simulink model "Model_compare_SLX"  (R2019b)
settings: Solver=VariableStepAuto  StartTime=0.0  StopTime=100.0  RelTol=1e-3
undefined symbols (not defined in the file): Ts, x0_dyn, x0_kin
settings Model: Creator=djtn  LastModifiedBy=alber
settings SFSimCC: CustomCodeUndefinedFunction=UseInterfaceOnly
settings ConfigComp: DVModelCoverageObjectives=MCDC  DVTestSuiteOptimization=Auto  DVDetectOutOfBounds=on  DVRebuildModelRepresentation=Always

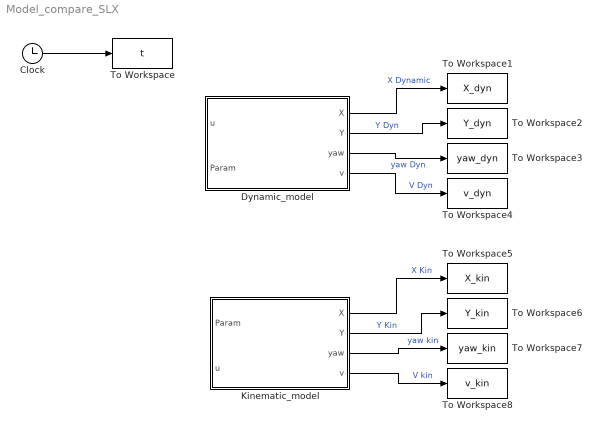
== system Model_compare_SLX ==
  Clock : Clock
  Dynamic_model : Subsystem
  Kinematic_model : Subsystem  TreatAsAtomicUnit=on
  To Workspace : ToWorkspace  VariableName=t  SampleTime=Ts
  To Workspace1 : ToWorkspace  VariableName=X_dyn  SampleTime=-1
  To Workspace2 : ToWorkspace  VariableName=Y_dyn  SampleTime=-1
  To Workspace3 : ToWorkspace  VariableName=yaw_dyn  SampleTime=-1
  To Workspace4 : ToWorkspace  VariableName=v_dyn  SampleTime=-1
  To Workspace5 : ToWorkspace  VariableName=X_kin  SampleTime=-1
  To Workspace6 : ToWorkspace  VariableName=Y_kin  SampleTime=-1
  To Workspace7 : ToWorkspace  VariableName=yaw_kin  SampleTime=-1
  To Workspace8 : ToWorkspace  VariableName=v_kin  SampleTime=-1
  wires:
  Clock/1 -> To Workspace/1
  Dynamic_model/1(X) -> To Workspace1/1  "X Dynamic"
  Dynamic_model/2(Y) -> To Workspace2/1  "Y Dyn"
  Dynamic_model/3(yaw) -> To Workspace3/1  "yaw Dyn"
  Dynamic_model/4(v) -> To Workspace4/1  "V Dyn"
  Kinematic_model/1(X) -> To Workspace5/1  "X Kin"
  Kinematic_model/2(Y) -> To Workspace6/1  "Y Kin"
  Kinematic_model/3(yaw) -> To Workspace7/1  "yaw kin"
  Kinematic_model/4(v) -> To Workspace8/1  "V kin"

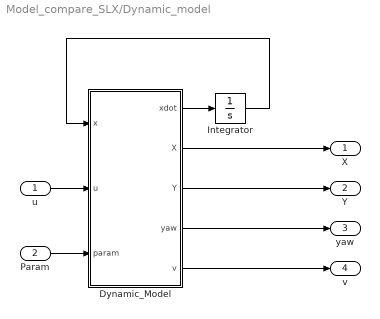
== system Model_compare_SLX/Dynamic_model ==
  u : Inport
  Param : Inport  Port=2
  Dynamic_Model : MATLAB Function  TreatAsAtomicUnit=on
  Integrator : Integrator  InitialCondition=x0_dyn
  X : Outport  PortDimensions=1  VectorParamsAs1DForOutWhenUnconnected=off
  Y : Outport  Port=2  PortDimensions=1  VectorParamsAs1DForOutWhenUnconnected=off
  yaw : Outport  Port=3  PortDimensions=1  VectorParamsAs1DForOutWhenUnconnected=off
  v : Outport  Port=4  PortDimensions=1  VectorParamsAs1DForOutWhenUnconnected=off
  wires:
  Integrator/1 -> Dynamic_Model/1(x)
  Dynamic_Model/1(xdot) -> Integrator/1
  u/1 -> Dynamic_Model/2(u)
  Dynamic_Model/2(X) -> X/1
  Dynamic_Model/3(Y) -> Y/1
  Dynamic_Model/4(yaw) -> yaw/1
  Dynamic_Model/5(v) -> v/1
  Param/1 -> Dynamic_Model/3(param)

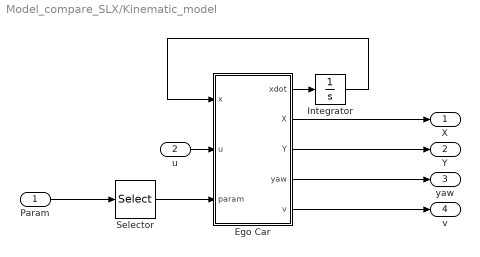
== system Model_compare_SLX/Kinematic_model ==
  Param : Inport
  u : Inport  Port=2
  Ego Car : MATLAB Function  TreatAsAtomicUnit=on
  Integrator : Integrator  InitialCondition=x0_kin
  Selector : Selector  InputPortWidth=6  IndexOptions=Index vector (dialog)  Indices=[1 2]  OutputSizes=1
  X : Outport  VectorParamsAs1DForOutWhenUnconnected=off
  Y : Outport  Port=2  VectorParamsAs1DForOutWhenUnconnected=off
  yaw : Outport  Port=3  VectorParamsAs1DForOutWhenUnconnected=off
  v : Outport  Port=4  VectorParamsAs1DForOutWhenUnconnected=off
  wires:
  Integrator/1 -> Ego Car/1(x)
  Ego Car/1(xdot) -> Integrator/1
  u/1 -> Ego Car/2(u)
  Ego Car/2(X) -> X/1
  Ego Car/3(Y) -> Y/1
  Ego Car/4(yaw) -> yaw/1
  Ego Car/5(v) -> v/1
  Param/1 -> Selector/1
  Selector/1 -> Ego Car/3(param)

== matlab function Model_compare_SLX/Dynamic_model/Dynamic_Model ==
  data: x input; u input; xdot output; param input; X output; Y output; yaw output; v output
function [xdot,X, Y, yaw, v] = fcn(x,u,param)

[xdot,X, Y, yaw, v] = VehicleModelCT_DYN(x,u,param);

== matlab function Model_compare_SLX/Kinematic_model/Ego Car ==
  settings: updateMethod=DISCRETE  sampleTime=Ts
  data: x input; u input; xdot output; X output; Y output; yaw output; v output; param input
function [xdot, X, Y, yaw, v] = fcn(x,u,param)
[xdot, X, Y, yaw, v] = obstacleVehicleModelCT(x,u,param);
